simulink model "testRotations"  (R2020a)
settings: Solver=VariableStepAuto  StartTime=0.0  StopTime=0  RelTol=1e-3
libraries: rotationAboutX x1, rotationAboutY x1, rotationAboutZ x1, rotationFromGroundToTangent x1, tangentialToGroundPosition x1
settings Model: Creator=Ayaz  LastModifiedBy=Ayaz

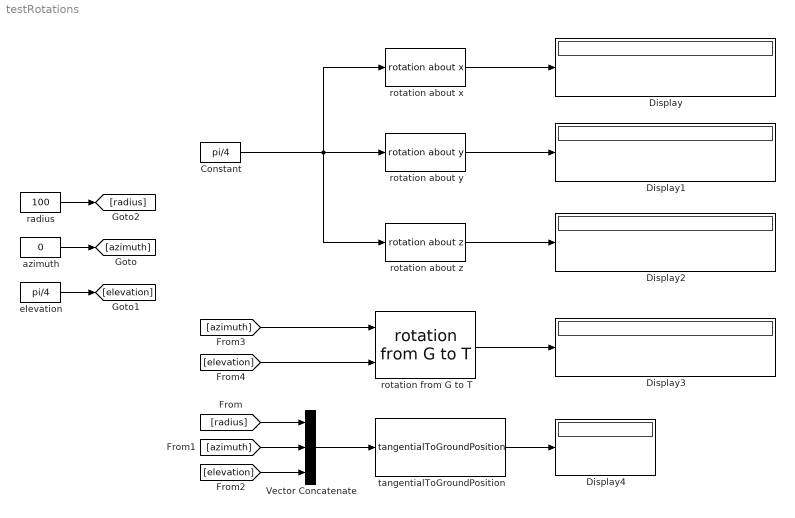
== system testRotations ==
  Constant : Constant  Value=pi/4  VectorParams1D=off
  Display{,1..4} (5 alike) : Display
  Vector Concatenate : Concatenate  NumInputs=3
  azimuth : Constant  Value=0  VectorParams1D=off
  elevation : Constant  Value=pi/4  VectorParams1D=off
  radius : Constant  Value=100
  rotation about x : rotationAboutX/rotation about x  SystemSampleTime=-1  Latency=0  AutoFrameSizeCalculation=off
  rotation about y : rotationAboutY/rotation about y  SystemSampleTime=-1  Latency=0  AutoFrameSizeCalculation=off
  rotation about z : rotationAboutZ/rotation about z  SystemSampleTime=-1  Latency=0  AutoFrameSizeCalculation=off
  rotation from G to T : rotationFromGroundToTangent/rotation from G to T  SystemSampleTime=-1  Latency=0  AutoFrameSizeCalculation=off
  tangentialToGroundPosition : tangentialToGroundPosition/tangentialToGroundPosition  SystemSampleTime=-1  Latency=0  AutoFrameSizeCalculation=off
  wires:
  Constant/1 -> rotation about z/1, rotation about x/1, rotation about y/1
  azimuth/1 -> [azimuth]
  elevation/1 -> [elevation]
  radius/1 -> [radius]
  [radius] -> Vector Concatenate/1
  [azimuth] -> Vector Concatenate/2
  [elevation] -> Vector Concatenate/3
  Vector Concatenate/1 -> tangentialToGroundPosition/1
  [azimuth] -> rotation from G to T/1
  [elevation] -> rotation from G to T/2
  rotation about x/1 -> Display/1
  rotation about y/1 -> Display1/1
  rotation about z/1 -> Display2/1
  rotation from G to T/1 -> Display3/1
  tangentialToGroundPosition/1 -> Display4/1
